simulink subsystem "lissajous_generator"  (R2019b)
settings: Solver=VariableStepAuto  StartTime=0.0  StopTime=10.0  RelTol=1e-3
libraries: quarc_library x4, SignalEditorBlockLib x1
settings Model: Creator=icpmoles  LastModifiedBy=icpmoles

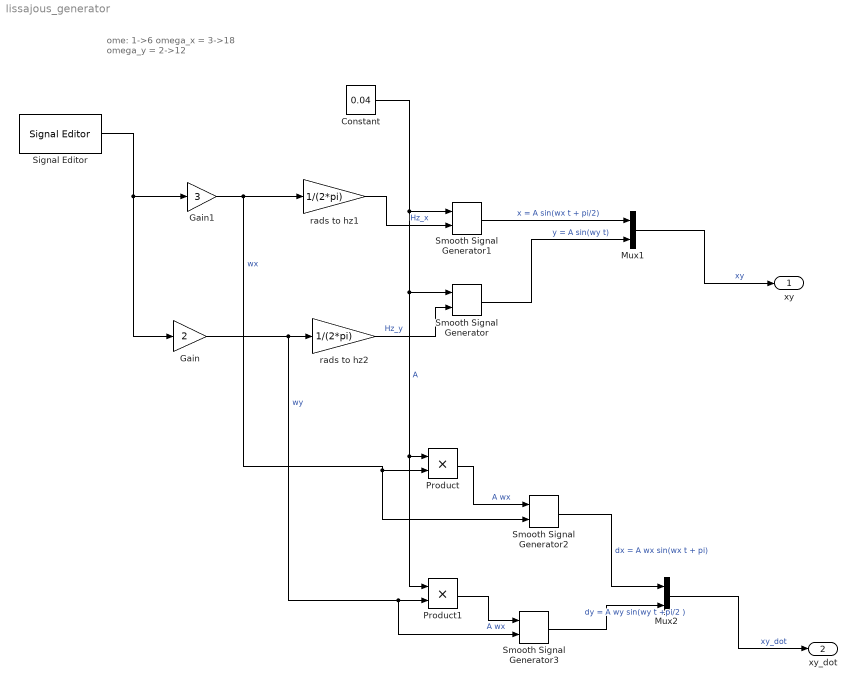
== system lissajous_generator ==
  note: ome: 1->6
      | omega_x = 3->18
      | omega_y = 2->12
  Constant : Constant  Value=0.04
  Gain : Gain  Gain=2
  Gain1 : Gain  Gain=3
  Mux1 : Mux  Inputs=2
  Mux2 : Mux  Inputs=2
  Product : Product
  Product1 : Product
  Signal Editor : SignalEditorBlockLib/Signal Editor  FileName=lissajous_base_omega.mat  ActiveScenario=liisajous  ActiveSignal=ome  IsBus=off  OutputBusObjectStr=Bus: BusObject  SampleTime=0  Interpolate=off  ZeroCross=off  OutputAfterFinalValue=Setting to zero  Unit=inherit  PreserveSignalName=on
      settings: SourceProductName=Simulink
  Smooth Signal Generator : quarc_library/Sources/Signals/Smooth Signal Generator  signal_type=Sine  source=External (input ports)  amplitude=1  frequency=1  initial_phase=0  sample_time=qc_get_step_size  output_cos=off
      settings: SourceProductName=QUARC Targets
  Smooth Signal Generator1 : quarc_library/Sources/Signals/Smooth Signal Generator  signal_type=Sine  source=External (input ports)  amplitude=1  frequency=1  initial_phase=pi/2  sample_time=qc_get_step_size  output_cos=off
      settings: SourceProductName=QUARC Targets
  Smooth Signal Generator2 : quarc_library/Sources/Signals/Smooth Signal Generator  signal_type=Sine  source=External (input ports)  amplitude=1  frequency=1  initial_phase=pi  sample_time=qc_get_step_size  output_cos=off
      settings: SourceProductName=QUARC Targets
  Smooth Signal Generator3 : quarc_library/Sources/Signals/Smooth Signal Generator  signal_type=Sine  source=External (input ports)  amplitude=1  frequency=1  initial_phase=pi/2  sample_time=qc_get_step_size  output_cos=off
      settings: SourceProductName=QUARC Targets
  rads to hz1 : Gain  Gain=1/(2*pi)
  rads to hz2 : Gain  Gain=1/(2*pi)
  xy : Outport
  xy_dot : Outport  Port=2
  wires:
  Gain/1 -> Smooth Signal Generator3/2, Product1/2, rads to hz2/1  "wy"
  Gain1/1 -> rads to hz1/1, Smooth Signal Generator2/2, Product/2  "wx"
  Product1/1 -> Smooth Signal Generator3/1  "A wx"
  rads to hz2/1 -> Smooth Signal Generator/2  "Hz_y"
  Smooth Signal Generator1/1 -> Mux1/1  "x = A sin(wx t + pi/2)"
  Smooth Signal Generator/1 -> Mux1/2  "y = A sin(wy t)"
  Signal Editor/1 -> Gain/1, Gain1/1
  Product/1 -> Smooth Signal Generator2/1  "A wx"
  Mux2/1 -> xy_dot/1  "xy_dot"
  Mux1/1 -> xy/1  "xy"
  Constant/1 -> Product1/1, Product/1, Smooth Signal Generator/1, Smooth Signal Generator1/1  "A"
  rads to hz1/1 -> Smooth Signal Generator1/2  "Hz_x"
  Smooth Signal Generator3/1 -> Mux2/2  "dy = A wy sin(wy t +pi/2 )"
  Smooth Signal Generator2/1 -> Mux2/1  "dx = A wx sin(wx t + pi)"
